simulink model "CanBusRagnar2020"  (R2021a)
settings: Solver=VariableStepAuto  StartTime=0.0  StopTime=10.0  RelTol=1e-3
model workspace (MAT data in the model file):
  A = [0  0  0  0  1  0  0  0; 0  0  0  0  0  1  0  0; 0  0  0  0  0  0  1  0; 0  0  0  0  0  0  0  1; 0  0  0  0  0  0  0  0; 0  0  0  0  0  0  0  0; 0  0  0  0  0  0  0  0; 0  0  0  0  0  0  0  0]
  Acl = [0  0  0  0  1  0  0  0  0  0  0  0  0  0  0  0; 0  0  0  0  0  1  0  0  0  0  0  0  0  0  0  0; 0  0  0  0  0  0  1  0  0  0  0  0  0  0  0  0; 0  0  0  0  0  0  0  1  0  0  0  0  0  0  0  0; 0  0  0  0  0  0  0  0  -1.14285714286  0  0  0  -2.14285714286  0  0  0; 0  0  0  0  0  0  0  0  0  -2.69387755102  0  0  0  -3.28571428571  0  0; 0  0  0  0  0  0  0  0  0  0  -2.38775510204  0  0  0  -3.14285714286  0; 0  0  0  0  0  0  0  0  0  0  0  -2.85714285714  0  0  0  -3.42857142857; 2  0  0  0  1  0  0  0  -2  0  0  0  0  0  0  0; 0  1.85714285714  0  0  0  1  0  0  0  -1.85714285714  0  0  0  0  0  0; 0  0  1.71428571429  0  0  0  1  0  0  0  -1.71428571429  0  0  0  0  0; 0  0  0  1.57142857143  0  0  0  1  0  0  0  -1.57142857143  0  0  0  0; 0  0  0  0  1.42857142857  0  0  0  -1.14285714286  0  0  0  -3.57142857143  0  0  0; 0  0  0  0  0  1.28571428571  0  0  0  -2.69387755102  0  0  0  -4.57142857143  0  0; 0  0  0  0  0  0  1.14285714286  0  0  0  -2.38775510204  0  0  0  -4.28571428571  0; 0  0  0  0  0  0  0  1  0  0  0  -2.85714285714  0  0  0  -4.42857142857]
  Aza = [-2  0  0  0  0  0  0  0; 0  -1.85714285714  0  0  0  0  0  0; 0  0  -1.71428571429  0  0  0  0  0; 0  0  0  -1.57142857143  0  0  0  0; -1.14285714286  0  0  0  -3.57142857143  0  0  0; 0  -2.69387755102  0  0  0  -4.57142857143  0  0; 0  0  -2.38775510204  0  0  0  -4.28571428571  0; 0  0  0  -2.85714285714  0  0  0  -4.42857142857]
  B = [0  0  0  0; 0  0  0  0; 0  0  0  0; 0  0  0  0; 0.78125  0  0  0; 0  0.78125  0  0; 0  0  0.78125  0; 0  0  0  2180]
  B_tilde_cl = [0  0  0  0; 0  0  0  0; 0  0  0  0; 0  0  0  0; 0.78125  0  0  0; 0  0.78125  0  0; 0  0  0.78125  0; 0  0  0  2180; 1.025390625  0  0  0; 0  0.0207149621212  0  0; 0  0  -0.0350560897436  0; 0  0  0  -81.75; 0.703125  0  0  0; 0  0.730298913043  0  0; 0  0  0.736860795455  0; 0  0  0  1703.125]
  C = [1  0  0  0  0  0  0  0; 0  1  0  0  0  0  0  0; 0  0  1  0  0  0  0  0; 0  0  0  1  0  0  0  0; 0  0  0  0  1  0  0  0; 0  0  0  0  0  1  0  0; 0  0  0  0  0  0  1  0; 0  0  0  0  0  0  0  1]
  Ccl = [1  0  0  0  0  0  0  0  0  0  0  0  0  0  0  0; 0  1  0  0  0  0  0  0  0  0  0  0  0  0  0  0; 0  0  1  0  0  0  0  0  0  0  0  0  0  0  0  0; 0  0  0  1  0  0  0  0  0  0  0  0  0  0  0  0; 0  0  0  0  1  0  0  0  0  0  0  0  0  0  0  0; 0  0  0  0  0  1  0  0  0  0  0  0  0  0  0  0; 0  0  0  0  0  0  1  0  0  0  0  0  0  0  0  0; 0  0  0  0  0  0  0  1  0  0  0  0  0  0  0  0]
  Cza = [1.46285714286  0  0  0  2.74285714286  0  0  0; 0  3.44816326531  0  0  0  4.20571428571  0  0; 0  0  3.05632653061  0  0  0  4.02285714286  0; 0  0  0  0.00131061598952  0  0  0  0.00157273918742]
  Desired_poles = [-2 -1.85714285714 -1.71428571429 -1.57142857143 -1.42857142857 -1.28571428571 -1.14285714286 -1]
  Desired_poles_obs = [-2 -1.85714285714 -1.71428571429 -1.57142857143 -1.42857142857 -1.28571428571 -1.14285714286 -1]
  Desired_zeroes = [-2 -1.85714285714 -1.71428571429 -1.57142857143 -1.42857142857 -1.28571428571 -1.14285714286 -1]
  F = [-1.46285714286  0  0  0  -2.74285714286  0  0  0; 0  -3.44816326531  0  0  0  -4.20571428571  0  0; 0  0  -3.05632653061  0  0  0  -4.02285714286  0; 0  0  0  -0.00131061598952  0  0  0  -0.00157273918742]
  F_mimo = [-1.46285714286  0  0  0  -2.74285714286  0  0  0; 0  -3.44816326531  0  0  0  -4.20571428571  0  0; 0  0  -3.05632653061  0  0  0  -4.02285714286  0; 0  0  0  -0.00131061598952  0  0  0  -0.00157273918742]
  L = [-2  0  0  0  -1  0  0  0; 0  -1.85714285714  0  0  0  -1  0  0; 0  0  -1.71428571429  0  0  0  -1  0; 0  0  0  -1.57142857143  0  0  0  -1; 0  0  0  0  -1.42857142857  0  0  0; 0  0  0  0  0  -1.28571428571  0  0; 0  0  0  0  0  0  -1.14285714286  0; 0  0  0  0  0  0  0  -1]
  L_mimo = [-2  0  0  0  -1  0  0  0; 0  -1.85714285714  0  0  0  -1  0  0; 0  0  -1.71428571429  0  0  0  -1  0; 0  0  0  -1.57142857143  0  0  0  -1; 0  0  0  0  -1.42857142857  0  0  0; 0  0  0  0  0  -1.28571428571  0  0; 0  0  0  0  0  0  -1.14285714286  0; 0  0  0  0  0  0  0  -1]
  M = [3.75  0  0  0  0  0  0  0; 0  0.0633116883117  0  0  0  0  0  0; 0  0  -0.0879120879121  0  0  0  0  0; 0  0  0  -0.0589285714286  0  0  0  0; 2.57142857143  0  0  0  0  0  0  0; 0  2.23203194321  0  0  0  0  0  0; 0  0  1.84786641929  0  0  0  0  0; 0  0  0  1.22767857143  0  0  0  0]
  M_tilde = [1.025390625  0  0  0; 0  0.0207149621212  0  0; 0  0  -0.0350560897436  0; 0  0  0  -81.75; 0.703125  0  0  0; 0  0.730298913043  0  0; 0  0  0.736860795455  0; 0  0  0  1703.125]
  N = [3.65714285714  0  0  0  0  0  0  0; 0  3.05632653061  0  0  0  0  0  0; 0  0  2.50775510204  0  0  0  0  0; 0  0  0  0.000720838794233  0  0  0  0]
  Sig = Simulink.Signal
  Sig.DataType = 'auto'
  Sig.Dimensions = -1
  Sig.DimensionsMode = 'auto'
  Sig.Complexity = 'auto'
  Sig.SampleTime = -1
  Sig.SamplingMode = 'auto'
  out = Simulink.SimulationOutput
  out.Data.tout = [0; 3.15544362088e-30; 0.005; 0.005; 0.005; 0.0050512; 0.0050512; 0.0050512; 0.0050512; 0.0051024; 0.0051024; 0.0051024; 0.0051536; 0.0051536; 0.0052048; 0.0052048; 0.005256; 0.005256; 0.005256; 0.0053072; 0.0053584; 0.0054608; 0.0056656; 0.0060752; 0.0068944; 0.00853279999999; 0.0100512; 0.0100512; 0.0101024; 0.0101024; 0.0101536; 0.0102048; 0.0103072; 0.010512; 0.0109216; 0.0117408; 0.0133792; 0.0151024; 0.0151024; 0.0183792; 0.0201024; 0.0201024; 0.0233792; 0.0251024; 0.0251024; 0.0283792; 0.031656; 0.0351024]
  out.Metadata = Simulink.SimulationMetadata
  out.Metadata.ModelInfo.ModelName = 'CanBusRagnar2020'
  out.Metadata.ModelInfo.ModelVersion = '2.7'
  out.Metadata.ModelInfo.ModelFilePath = 'C:\Users\mozzr\Documents\control-courses\TrueTime_Ragnar_TaskSpace_Observer\CanBusRagnar2020.slx'
  out.Metadata.ModelInfo.UserID = 'mozzr'
  out.Metadata.ModelInfo.MachineName = 'DESKTOP-FJO0ONK'
  out.Metadata.ModelInfo.Platform = 'PCWIN64'
  out.Metadata.ModelInfo.ModelStructuralChecksum = [3509124868; 2074894372; 1704497093; 2226183946]
  out.Metadata.ModelInfo.SimulationMode = 'normal'
  out.Metadata.ModelInfo.StartTime = 0
  out.Metadata.ModelInfo.StopTime = 0.0351024
  out.Metadata.ModelInfo.SolverInfo.Type = 'Variable-Step'
  out.Metadata.ModelInfo.SolverInfo.Solver = 'ode45'
  out.Metadata.ModelInfo.SolverInfo.MaxStepSize = 0.2
  out.Metadata.ModelInfo.SimulinkVersion.Name = 'Simulink'
  out.Metadata.ModelInfo.SimulinkVersion.Version = '10.3'
  out.Metadata.ModelInfo.SimulinkVersion.Release = '(R2021a)'
  out.Metadata.ModelInfo.SimulinkVersion.Date = '14-Nov-2020'
  out.Metadata.ModelInfo.LoggingInfo.LoggingToFile = 'off'
  out.Metadata.TimingInfo.WallClockTimestampStart = '2021-11-12 14:45:38'
  out.Metadata.TimingInfo.WallClockTimestampStop = '2021-11-12 14:45:41'
  out.Metadata.TimingInfo.InitializationElapsedWallTime = 1.9336621
  out.Metadata.TimingInfo.ExecutionElapsedWallTime = 0.310442
  out.Metadata.TimingInfo.TerminationElapsedWallTime = 0.0323667
  out.Metadata.TimingInfo.TotalElapsedWallTime = 2.2764708
  out.Metadata.TimingInfo.ProfilerData = 'Profiler is not enabled'
  out.Metadata.ExecutionInfo.StopEvent = 'DiagnosticError'
  out.Metadata.ExecutionInfo.StopEventSource = []
  out.Metadata.ExecutionInfo.StopEventDescription = 'Error occurred in ''<a href="matlab:open_and_hilite_hyperlink (''CanBusRagnar2020/TrueTime Kernel (Teensy)'',''error'')">CanBusRagnar2020/TrueTime Kernel (Teensy)</a>''. Unrecognized function or variable ''A''.'
  out.Metadata.ExecutionInfo.ErrorDiagnostic.Diagnostic = MSLDiagnostic
  out.Metadata.ExecutionInfo.ErrorDiagnostic.Diagnostic.identifier = 'Simulink:blocks:SubsysErrFcnMsg'
  out.Metadata.ExecutionInfo.ErrorDiagnostic.Diagnostic.message = 'Error occurred in ''<a href="matlab:open_and_hilite_hyperlink (''CanBusRagnar2020/TrueTime Kernel (Teensy)'',''error'')">CanBusRagnar2020/TrueTime Kernel (Teensy)</a>''. Unrecognized function or variable ''A''.'
  out.Metadata.ExecutionInfo.ErrorDiagnostic.Diagnostic.paths = {'CanBusRagnar2020/TrueTime Kernel (Teensy)'}
  out.Metadata.ExecutionInfo.ErrorDiagnostic.Diagnostic.cause{1} = MSLDiagnostic
  out.Metadata.ExecutionInfo.ErrorDiagnostic.Diagnostic.cause{1}.identifier = 'Simulink:blocks:SubsysErrFcnMsg'
  out.Metadata.ExecutionInfo.ErrorDiagnostic.Diagnostic.cause{1}.message = 'Error occurred in ''CanBusRagnar2020/TrueTime Kernel (Teensy)''. Unrecognized function or variable ''A''.'
  out.Metadata.ExecutionInfo.ErrorDiagnostic.Diagnostic.cause{1}.paths = {'CanBusRagnar2020/TrueTime Kernel (Teensy)'}
  out.Metadata.ExecutionInfo.ErrorDiagnostic.Diagnostic.cause{1}.arguments = {'CanBusRagnar2020/TrueTime Kernel (Teensy)', 'Unrecognized function or variable ''A''.'}
  out.Metadata.ExecutionInfo.ErrorDiagnostic.Diagnostic.cause{1}.stack = struct([])
  out.Metadata.ExecutionInfo.ErrorDiagnostic.Diagnostic.cause{1}.metaDataProp.UI = []
  out.Metadata.ExecutionInfo.ErrorDiagnostic.Diagnostic.cause{1}.metaDataProp.STAGE = []
  out.Metadata.ExecutionInfo.ErrorDiagnostic.Diagnostic.cause{1}.metaDataProp.CATEGORY = []
  out.Metadata.ExecutionInfo.ErrorDiagnostic.Diagnostic.cause{1}.metaDataProp.COMPONENT = []
  out.Metadata.ExecutionInfo.ErrorDiagnostic.Diagnostic.cause{1}.metaDataProp.MDL_NAME = []
  out.Metadata.ExecutionInfo.ErrorDiagnostic.Diagnostic.cause{1}.metaDataProp.ACTION = ''
  out.Metadata.ExecutionInfo.ErrorDiagnostic.Diagnostic.cause{1}.metaDataProp.DOC = []
  out.Metadata.ExecutionInfo.ErrorDiagnostic.Diagnostic.cause{1}.metaDataProp.SUB_CATEGORY = []
  out.Metadata.ExecutionInfo.ErrorDiagnostic.Diagnostic.cause{1}.metaDataProp.MSTACK_PRESERVE = []
  out.Metadata.ExecutionInfo.ErrorDiagnostic.Diagnostic.cause{1}.metaDataProp.DOUBLE_ARGS = []
  out.Metadata.ExecutionInfo.ErrorDiagnostic.Diagnostic.arguments = {'CanBusRagnar2020/TrueTime Kernel (Teensy)', 'Unrecognized function or variable ''A''.'}
  out.Metadata.ExecutionInfo.ErrorDiagnostic.Diagnostic.stack = struct([])
  out.Metadata.ExecutionInfo.ErrorDiagnostic.Diagnostic.metaDataProp.UI = []
  out.Metadata.ExecutionInfo.ErrorDiagnostic.Diagnostic.metaDataProp.STAGE = []
  out.Metadata.ExecutionInfo.ErrorDiagnostic.Diagnostic.metaDataProp.CATEGORY = []
  out.Metadata.ExecutionInfo.ErrorDiagnostic.Diagnostic.metaDataProp.COMPONENT = []
  out.Metadata.ExecutionInfo.ErrorDiagnostic.Diagnostic.metaDataProp.MDL_NAME = []
  out.Metadata.ExecutionInfo.ErrorDiagnostic.Diagnostic.metaDataProp.ACTION = ''
  out.Metadata.ExecutionInfo.ErrorDiagnostic.Diagnostic.metaDataProp.DOC = []
  out.Metadata.ExecutionInfo.ErrorDiagnostic.Diagnostic.metaDataProp.SUB_CATEGORY = []
  out.Metadata.ExecutionInfo.ErrorDiagnostic.Diagnostic.metaDataProp.MSTACK_PRESERVE = []
  out.Metadata.ExecutionInfo.ErrorDiagnostic.Diagnostic.metaDataProp.DOUBLE_ARGS = []
  out.Metadata.ExecutionInfo.ErrorDiagnostic.SimulationPhase = 'Execution'
  out.Metadata.ExecutionInfo.ErrorDiagnostic.SimulationTime = 0.0351024
  out.Metadata.ExecutionInfo.WarningDiagnostics = struct([])
  out.Metadata.AppInfo = struct()
  out.ErrorMessage = 'Error occurred in ''<a href="matlab:open_and_hilite_hyperlink (''CanBusRagnar2020/TrueTime Kernel (Teensy)'',''error'')">CanBusRagnar2020/TrueTime Kernel (Teensy)</a>''. Unrecognized function or variable ''A''.
    | Caused by:
    |     Error occurred in ''CanBusRagnar2020/TrueTime Kernel (Teensy)''. Unrecognized function or variable ''A''.'
  ref = [0.01 0.51 -0.41 1.4835298642 0 0 0 0]
  sys_mimo = ss
  sys_mimo.IOSize_ = [8 4]
  sys_mimo.Data_ = ltipack.ssdata
  sys_mimo.Data_.a = [0  0  0  0  1  0  0  0; 0  0  0  0  0  1  0  0; 0  0  0  0  0  0  1  0; 0  0  0  0  0  0  0  1; 0  0  0  0  0  0  0  0; 0  0  0  0  0  0  0  0; 0  0  0  0  0  0  0  0; 0  0  0  0  0  0  0  0]
  sys_mimo.Data_.b = [0  0  0  0; 0  0  0  0; 0  0  0  0; 0  0  0  0; 0.78125  0  0  0; 0  0.78125  0  0; 0  0  0.78125  0; 0  0  0  2180]
  sys_mimo.Data_.c = [1  0  0  0  0  0  0  0; 0  1  0  0  0  0  0  0; 0  0  1  0  0  0  0  0; 0  0  0  1  0  0  0  0; 0  0  0  0  1  0  0  0; 0  0  0  0  0  1  0  0; 0  0  0  0  0  0  1  0; 0  0  0  0  0  0  0  1]
  sys_mimo.Data_.d = [0  0  0  0; 0  0  0  0; 0  0  0  0; 0  0  0  0; 0  0  0  0; 0  0  0  0; 0  0  0  0; 0  0  0  0]
  sys_mimo.Data_.Delay.Input = [0; 0; 0; 0]
  sys_mimo.Data_.Delay.Output = [0; 0; 0; 0; 0; 0; 0; 0]
  sys_mimo.Data_.Delay.Internal = []
  sys_mimo.Data_.Ts = 0
values from neighbouring files (symbols this model uses):
  sys_mimo = ss(A,B,C,0)    [SS_MIMO.m]
libraries: truetime x6
settings Model: Creator=mozzr  LastModifiedBy=mozzr
settings SolverCC: AlgebraicLoopSolver=TrustRegion

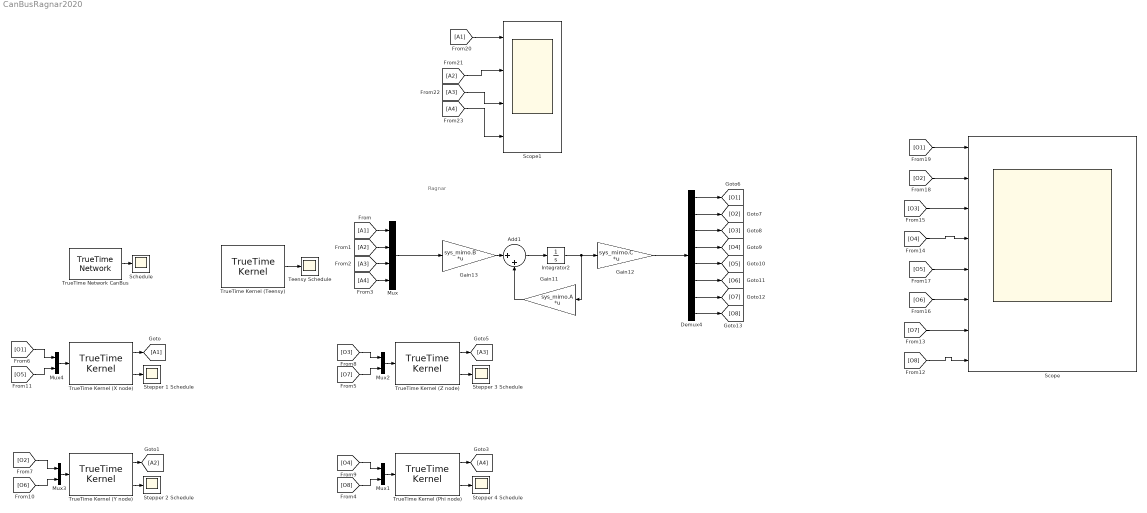
== system CanBusRagnar2020 ==
  note: Ragnar
  Add1 : Sum  Inputs=|++
  Demux4 : Demux  Outputs=8
  Gain11 : Gain  Gain=sys_mimo.A  Multiplication=Matrix(K*u)
  Gain12 : Gain  Gain=sys_mimo.C  Multiplication=Matrix(K*u)
  Gain13 : Gain  Gain=sys_mimo.B  Multiplication=Matrix(K*u)
  Integrator2 : Integrator  InitialCondition=[0 0.5 -0.4 deg2rad(90) 0 0 0 0]
  Mux : Mux
  Mux{1..4} (4 alike) : Mux  Inputs=2
  Schedule : Scope
  Scope : Scope  NumInputPorts=8
  Scope1 : Scope  NumInputPorts=4
  Stepper 1 Schedule : Scope
  Stepper 2 Schedule : Scope
  Stepper 3 Schedule : Scope
  Stepper 4 Schedule : Scope
  Teensy Schedule : Scope
  TrueTime Kernel (Phi node) : truetime/TrueTime Kernel  sfun=nodePhi_init  args=[]  ninputsoutputs=[2 1]  ntriggers=0  trigtype=falling  nwnodenbr=[1 5]  clockoffsetdrift=[0 0]  schedoutput=on  battery=off  poweroutput=off  label=1: 5
  TrueTime Kernel (Teensy) : truetime/TrueTime Kernel  sfun=Teensy_init  args=[]  ninputsoutputs=[0 0]  ntriggers=0  trigtype=falling  nwnodenbr=[1 1]  clockoffsetdrift=[0 0]  schedoutput=on  battery=off  poweroutput=off  label=1: 1
  TrueTime Kernel (X node) : truetime/TrueTime Kernel  sfun=nodeX_init  args=[]  ninputsoutputs=[2 1]  ntriggers=0  trigtype=falling  nwnodenbr=[1 2]  clockoffsetdrift=[0 0]  schedoutput=on  battery=off  poweroutput=off  label=1: 2
  TrueTime Kernel (Y node) : truetime/TrueTime Kernel  sfun=nodeY_init  args=[]  ninputsoutputs=[2 1]  ntriggers=0  trigtype=falling  nwnodenbr=[1 3]  clockoffsetdrift=[0 0]  schedoutput=on  battery=off  poweroutput=off  label=1: 3
  TrueTime Kernel (Z node) : truetime/TrueTime Kernel  sfun=nodeZ_init  args=[]  ninputsoutputs=[2 1]  ntriggers=0  trigtype=falling  nwnodenbr=[1 4]  clockoffsetdrift=[0 0]  schedoutput=on  battery=off  poweroutput=off  label=1: 4
  TrueTime Network CanBus : truetime/TrueTime Network  nwtype=CSMA/AMP (CAN)  nwnbr=1  nnodes=5  rate=10000000  minsize=512  lossprob=0  seed=0  bandwidths=[0.5 0.5]  slotsize=512  schedule=[1 1 2]  memsize=80000  buftype=Common buffer  overflow=Retransmit  dynSchedule=0  miniSlotSize=0  NIT=0  QSortMode=FIFO  sync=0  irtSchedule=0  nrtLength=0  nodeGraph=0  scheduleoutput=on
  wires:
  TrueTime Kernel (Y node)/2 -> Stepper 2 Schedule/1
  TrueTime Kernel (X node)/2 -> Stepper 1 Schedule/1
  TrueTime Kernel (Phi node)/2 -> Stepper 4 Schedule/1
  TrueTime Kernel (Z node)/2 -> Stepper 3 Schedule/1
  TrueTime Kernel (Teensy)/1 -> Teensy Schedule/1
  TrueTime Network CanBus/1 -> Schedule/1
  TrueTime Kernel (X node)/1 -> [A1]
  [A1] -> Mux/1
  TrueTime Kernel (Y node)/1 -> [A2]
  TrueTime Kernel (Phi node)/1 -> [A4]
  TrueTime Kernel (Z node)/1 -> [A3]
  [A2] -> Mux/2
  [A3] -> Mux/3
  [A4] -> Mux/4
  Demux4/1 -> [O1]
  Demux4/2 -> [O2]
  Demux4/3 -> [O3]
  Demux4/4 -> [O4]
  Demux4/5 -> [O5]
  Demux4/6 -> [O6]
  Demux4/7 -> [O7]
  Demux4/8 -> [O8]
  Mux1/1 -> TrueTime Kernel (Phi node)/1
  [O4] -> Mux1/1
  [O8] -> Mux1/2
  [O3] -> Mux2/1
  [O7] -> Mux2/2
  Mux2/1 -> TrueTime Kernel (Z node)/1
  [O2] -> Mux3/1
  [O6] -> Mux3/2
  Mux3/1 -> TrueTime Kernel (Y node)/1
  [O1] -> Mux4/1
  [O5] -> Mux4/2
  Mux4/1 -> TrueTime Kernel (X node)/1
  Gain11/1 -> Add1/2
  Gain13/1 -> Add1/1
  Add1/1 -> Integrator2/1
  Mux/1 -> Gain13/1
  Integrator2/1 -> Gain11/1, Gain12/1
  Gain12/1 -> Demux4/1
  [O8] -> Scope/8
  [O7] -> Scope/7
  [O4] -> Scope/4
  [O3] -> Scope/3
  [O5] -> Scope/5
  [O6] -> Scope/6
  [O2] -> Scope/2
  [O1] -> Scope/1
  [A1] -> Scope1/1
  [A2] -> Scope1/2
  [A3] -> Scope1/3
  [A4] -> Scope1/4
